simulink model "fulladder"  (R2025b)
settings: Solver=VariableStepAuto  StartTime=0.0  StopTime=10.0  RelTol=1e-3
settings Model: Creator=cyber  LastModifiedBy=cyber

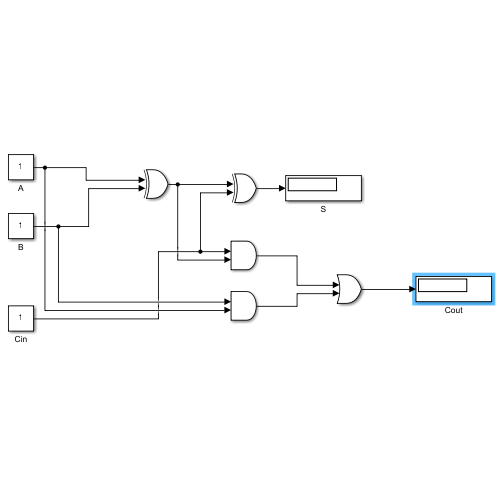
[thumbnail: Simulink's stored preview of the top-level diagram]
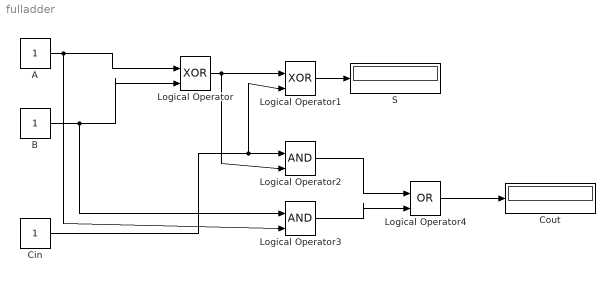
== system fulladder ==
  A : Constant
  B : Constant
  Cin : Constant
  Cout : Display
  Logical Operator : Logic  Operator=XOR  IconShape=distinctive  AllPortsSameDT=off  OutDataTypeStr=boolean
  Logical Operator1 : Logic  Operator=XOR  IconShape=distinctive  AllPortsSameDT=off  OutDataTypeStr=boolean
  Logical Operator2 : Logic  IconShape=distinctive  AllPortsSameDT=off  OutDataTypeStr=boolean
  Logical Operator3 : Logic  IconShape=distinctive  AllPortsSameDT=off  OutDataTypeStr=boolean
  Logical Operator4 : Logic  Operator=OR  IconShape=distinctive  AllPortsSameDT=off  OutDataTypeStr=boolean
  S : Display
  wires:
  A/1 -> Logical Operator3/2, Logical Operator/1
  B/1 -> Logical Operator3/1, Logical Operator/2
  Logical Operator/1 -> Logical Operator2/2, Logical Operator1/1
  Cin/1 -> Logical Operator2/1, Logical Operator1/2
  Logical Operator2/1 -> Logical Operator4/1
  Logical Operator3/1 -> Logical Operator4/2
  Logical Operator1/1 -> S/1
  Logical Operator4/1 -> Cout/1
